simulink model "simulink_coder_extrinsic"  (R2023a)
settings: Solver=VariableStepAuto  StartTime=0.0  StopTime=20  RelTol=1e-3
settings Model: Creator=zoufi  LastModifiedBy=zoufi

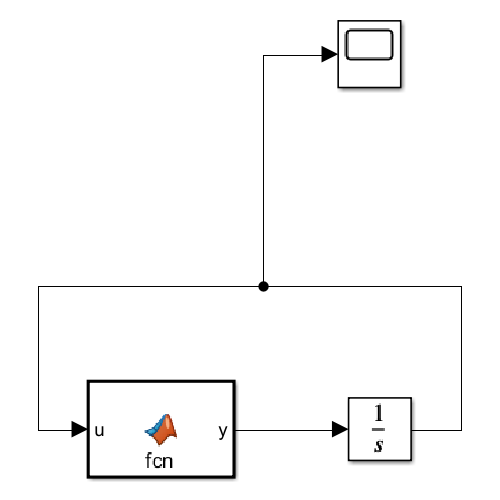
[thumbnail: Simulink's stored preview of the top-level diagram]
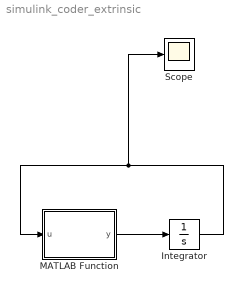
== system simulink_coder_extrinsic ==
  Integrator : Integrator  InitialCondition=[2; 0]
  MATLAB Function : MATLAB Function  TreatAsAtomicUnit=on
  Scope : Scope
  wires:
  MATLAB Function/1(y) -> Integrator/1
  Integrator/1 -> Scope/1, MATLAB Function/1(u)

== matlab function simulink_coder_extrinsic/MATLAB Function ==
  data: u input; y output
function y = fcn(u)
coder.extrinsic("myfun.m")
y = myfun(0,u);
